simulink model "Mod_No_Lineal"  (R2020b)
settings: Solver=VariableStepAuto  StartTime=0.0  StopTime=10.0  RelTol=1e-3
undefined symbols (not defined in the file): AC, I, K, mgL, PWM
settings Model: Creator=andre  LastModifiedBy=andre

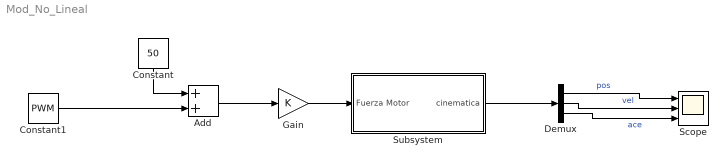
== system Mod_No_Lineal ==
  Add : Sum
  Constant : Constant  Value=50
  Constant1 : Constant  Value=PWM
  Demux : Demux  Outputs=3
  Gain : Gain  Gain=K
  Scope : Scope  NumInputPorts=3
  Subsystem : Subsystem
  wires:
  Gain/1 -> Subsystem/1(Fuerza Motor)
  Constant/1 -> Add/1
  Add/1 -> Gain/1
  Constant1/1 -> Add/2
  Subsystem/1(cinematica) -> Demux/1
  Demux/1 -> Scope/1  "pos"
  Demux/2 -> Scope/2  "vel"
  Demux/3 -> Scope/3  "ace"

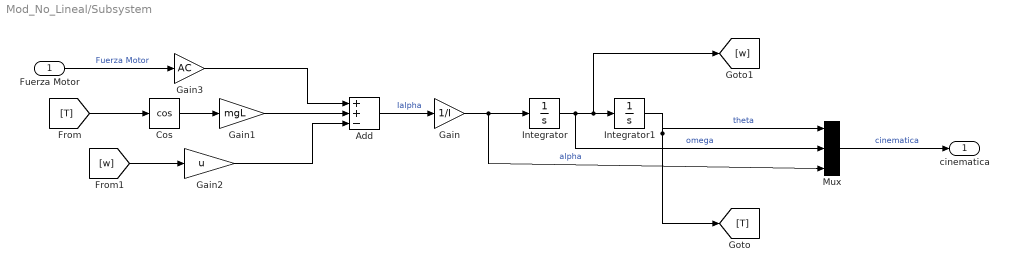
== system Mod_No_Lineal/Subsystem ==
  Fuerza Motor : Inport
  Add : Sum  Inputs=++-
  Cos : Trigonometry  Operator=cos
  Gain : Gain  Gain=1/I
  Gain1 : Gain  Gain=mgL
  Gain2 : Gain  Gain=u
  Gain3 : Gain  Gain=AC
  Integrator : Integrator
  Integrator1 : Integrator  InitialCondition=-70
  Mux : Mux  Inputs=3
  cinematica : Outport
  wires:
  Add/1 -> Gain/1  "Ialpha"
  Gain2/1 -> Add/3
  Integrator1/1 -> [T], Mux/1  "theta"
  Integrator/1 -> Mux/2, [w], Integrator1/1  "omega"
  Cos/1 -> Gain1/1
  Gain/1 -> Mux/3, Integrator/1  "alpha"
  Gain3/1 -> Add/1
  [w] -> Gain2/1
  Gain1/1 -> Add/2
  [T] -> Cos/1
  Mux/1 -> cinematica/1  "cinematica"
  Fuerza Motor/1 -> Gain3/1  "Fuerza Motor"
